simulink library "dsc"  (R2021b)
settings: Solver=VariableStepAuto  StartTime=0.0  StopTime=10.0  RelTol=1e-3
undefined symbols (not defined in the file): DEG2RAD, ENUM_DISCSTA_ACTIVE, ENUM_DISCSTA_Disabled, ENUM_DISCSTA_OFF, ENUM_DISCSTA_STANDBY, FALSE, KDSC_AccPedalOvrd_flg, KDSC_ActiveAllowTime_s, KDSC_BrkDisBand_pct, KDSC_BrkEnBand_pct, KDSC_BrkPedalOvrd_flg, KDSC_CGRealAxle_m, KDSC_FirstOrderInpTs_s, KDSC_LongAccelLimit_g, KDSC_MaxSpeed_kph, KDSC_MinSpeed_kph, KDSC_SamplingTime_s, KDSC_SpdRangeHigh_kph, KDSC_SpdRangeLow_kph, KDSC_TriggerTimes, KDSC_TurnAngControlpoint1_deg, KDSC_TurnAngControlpoint1_kph, KDSC_TurnAngControlpoint2_deg, KDSC_TurnAngControlpoint2_kph, KDSC_TurnAngExit_deg, KDSC_TurnAngLimit_deg, KINP_DISCButtReq_flg_ovrdflg, KINP_DISCButtReq_flg_ovrdval, RAD2DEG, TRUE, ZERO_FLOAT
libraries: simulink x13, hcu_lib x2
settings Model: Creator=FVT22120  LastModifiedBy=FVT23010

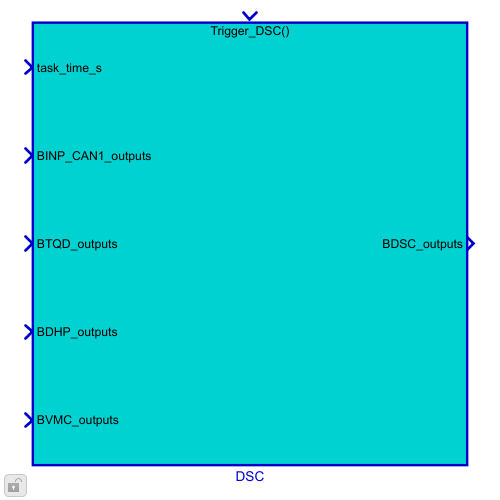
[thumbnail: Simulink's stored preview of the top-level diagram]
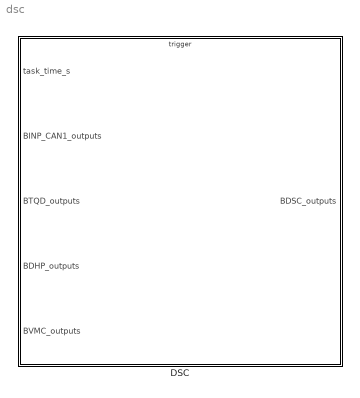
== system dsc ==
  DSC : Subsystem
      settings: RTWSystemCode=Nonreusable function  RTWFcnNameOpts=Use subsystem name  RTWFileNameOpts=Use subsystem name

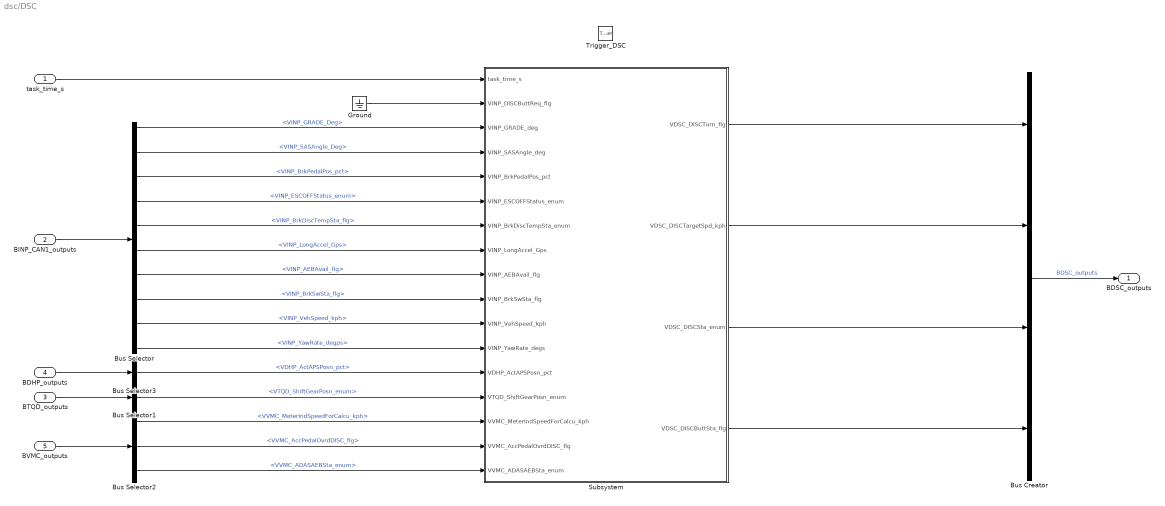
== system dsc/DSC ==
  task_time_s : Inport
  BINP_CAN1_outputs : Inport  Port=2  OutDataTypeStr=Bus: BINP_CAN1_outputs
  BTQD_outputs : Inport  Port=3  OutDataTypeStr=Bus: BTQD_outputs
  BDHP_outputs : Inport  Port=4  OutDataTypeStr=Bus: BDHP_outputs
  BVMC_outputs : Inport  Port=5  OutDataTypeStr=Bus: BVMC_outputs
  Trigger_DSC : TriggerPort  TriggerType=function-call  VariantControl=(inherit)  PortDimensions=1
  Bus Creator : BusCreator  Inputs=4  OutDataTypeStr=Bus: BDSC_outputs  NonVirtualBus=on
  Bus Selector : BusSelector  OutputSignals=VINP_GRADE_Deg,VINP_SASAngle_Deg,VINP_BrkPedalPos_pct,VINP_ESCOFFStatus_enum,VINP_BrkDiscTempSta_flg,VINP_LongAccel_Gps,VINP_AEBAvail_flg,VINP_BrkSwSta_flg,VINP_VehSpeed_kph,VINP_YawRate_degps
  Bus Selector1 : BusSelector  OutputSignals=VTQD_ShiftGearPosn_enum
  Bus Selector2 : BusSelector  OutputSignals=VVMC_MeterIndSpeedForCalcu_kph,VVMC_AccPedalOvrdDISC_flg,VVMC_ADASAEBSta_enum
  Bus Selector3 : BusSelector  OutputSignals=VDHP_ActAPSPosn_pct
  Ground : Ground
  Subsystem : Subsystem
  BDSC_outputs : Outport  OutDataTypeStr=Bus: BDSC_outputs
  wires:
  Bus Creator/1 -> BDSC_outputs/1  "BDSC_outputs"
  BINP_CAN1_outputs/1 -> Bus Selector/1
  BTQD_outputs/1 -> Bus Selector1/1
  BDHP_outputs/1 -> Bus Selector3/1
  task_time_s/1 -> Subsystem/1(task_time_s)
  Ground/1 -> Subsystem/2(VINP_DISCButtReq_flg)
  Bus Selector2/3 -> Subsystem/17(VVMC_ADASAEBSta_enum)  "<VVMC_ADASAEBSta_enum>"
  Bus Selector1/1 -> Subsystem/14(VTQD_ShiftGearPosn_enum)  "<VTQD_ShiftGearPosn_enum>"
  Bus Selector3/1 -> Subsystem/13(VDHP_ActAPSPosn_pct)  "<VDHP_ActAPSPosn_pct>"
  Subsystem/1(VDSC_DISCTurn_flg) -> Bus Creator/1
  Subsystem/2(VDSC_DISCTargetSpd_kph) -> Bus Creator/2
  Subsystem/3(VDSC_DISCSta_enum) -> Bus Creator/3
  Subsystem/4(VDSC_DISCButtSta_flg) -> Bus Creator/4
  BVMC_outputs/1 -> Bus Selector2/1
  Bus Selector2/1 -> Subsystem/15(VVMC_MeterIndSpeedForCalcu_kph)  "<VVMC_MeterIndSpeedForCalcu_kph>"
  Bus Selector2/2 -> Subsystem/16(VVMC_AccPedalOvrdDISC_flg)  "<VVMC_AccPedalOvrdDISC_flg>"
  Bus Selector/1 -> Subsystem/3(VINP_GRADE_deg)  "<VINP_GRADE_Deg>"
  Bus Selector/2 -> Subsystem/4(VINP_SASAngle_deg)  "<VINP_SASAngle_Deg>"
  Bus Selector/3 -> Subsystem/5(VINP_BrkPedalPos_pct)  "<VINP_BrkPedalPos_pct>"
  Bus Selector/4 -> Subsystem/6(VINP_ESCOFFStatus_enum)  "<VINP_ESCOFFStatus_enum>"
  Bus Selector/5 -> Subsystem/7(VINP_BrkDiscTempSta_enum)  "<VINP_BrkDiscTempSta_flg>"
  Bus Selector/6 -> Subsystem/8(VINP_LongAccel_Gps)  "<VINP_LongAccel_Gps>"
  Bus Selector/7 -> Subsystem/9(VINP_AEBAvail_flg)  "<VINP_AEBAvail_flg>"
  Bus Selector/8 -> Subsystem/10(VINP_BrkSwSta_flg)  "<VINP_BrkSwSta_flg>"
  Bus Selector/9 -> Subsystem/11(VINP_VehSpeed_kph)  "<VINP_VehSpeed_kph>"
  Bus Selector/10 -> Subsystem/12(VINP_YawRate_degs)  "<VINP_YawRate_degps>"

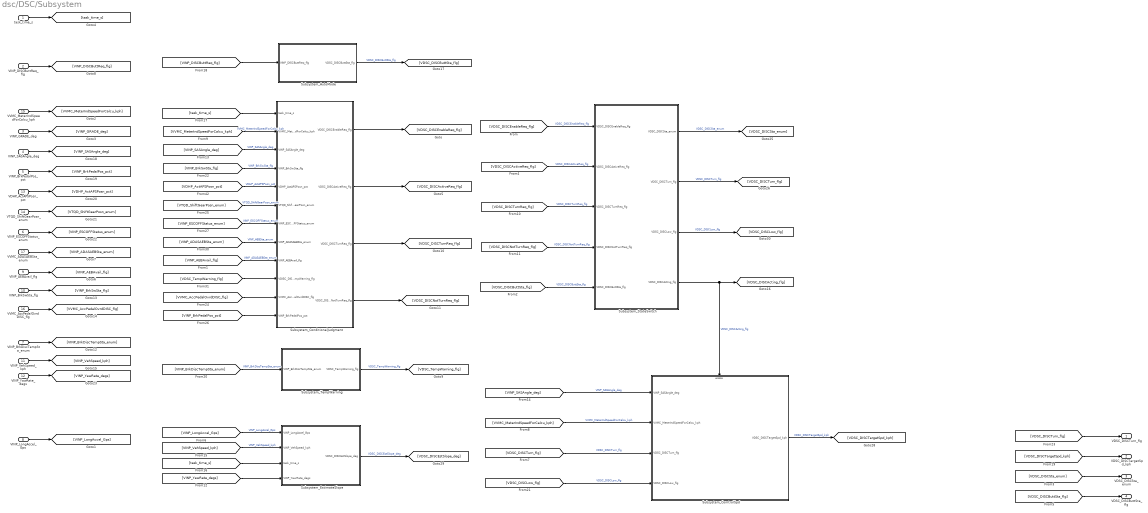
== system dsc/DSC/Subsystem ==
  task_time_s : Inport
  VINP_DISCButtReq_flg : Inport  Port=2
  VINP_GRADE_deg : Inport  Port=3
  VINP_SASAngle_deg : Inport  Port=4
  VINP_BrkPedalPos_pct : Inport  Port=5
  VINP_ESCOFFStatus_enum : Inport  Port=6
  VINP_BrkDiscTempSta_enum : Inport  Port=7
  VINP_LongAccel_Gps : Inport  Port=8
  VINP_AEBAvail_flg : Inport  Port=9
  VINP_BrkSwSta_flg : Inport  Port=10
  VINP_VehSpeed_kph : Inport  Port=11
  VINP_YawRate_degs : Inport  Port=12
  VDHP_ActAPSPosn_pct : Inport  Port=13
  VTQD_ShiftGearPosn_enum : Inport  Port=14
  VVMC_MeterIndSpeedForCalcu_kph : Inport  Port=15
  VVMC_AccPedalOvrdDISC_flg : Inport  Port=16
  VVMC_ADASAEBSta_enum : Inport  Port=17
  Subsystem_AutoMode : Subsystem
  Subsystem_ComtrolSpd : Subsystem  TreatAsAtomicUnit=on
  Subsystem_ConditionalJudgment : Subsystem
  Subsystem_EstimateSlope : Subsystem
  Subsystem_StateSwitch : Subsystem
  Subsystem_TempWarning : Subsystem
  VDSC_DISCTurn_flg : Outport
  VDSC_DISCTargetSpd_kph : Outport  Port=2
  VDSC_DISCSta_enum : Outport  Port=3
  VDSC_DISCButtSta_flg : Outport  Port=4
  wires:
  Subsystem_StateSwitch/4(VDSC_DISCActing_flg) -> [VDSC_DISCActing_flg], Subsystem_ComtrolSpd/Enable  "VDSC_DISCActing_flg"
  [VINP_SASAngle_deg] -> Subsystem_ConditionalJudgment/3("VINP_SASAngle_deg ")  "VINP_SASAngle_deg"
  [VDSC_DISCEnableReq_flg] -> Subsystem_StateSwitch/1(VDSC_DISCEnableReq_flg)  "VDSC_DISCEnableReq_flg"
  Subsystem_StateSwitch/2(VDSC_DISCTurn_flg) -> [VDSC_DISCTurn_flg]  "VDSC_DISCTurn_flg"
  [VINP_VehSpeed_kph] -> Subsystem_EstimateSlope/2(VINP_VehSpeed_kph)  "VINP_VehSpeed_kph"
  [VINP_DISCButtReq_flg] -> Subsystem_AutoMode/1(VINP_DISCButtReq_flg)
  VINP_GRADE_deg/1 -> [VINP_GRADE_deg]
  Subsystem_EstimateSlope/1(VDSC_DISCEstSlope_deg) -> [VDSC_DISCEstSlope_deg]  "VDSC_DISCEstSlope_deg"
  VTQD_ShiftGearPosn_enum/1 -> [VTQD_ShiftGearPosn_enum]
  Subsystem_ConditionalJudgment/3(VDSC_DISCTurnReq_flg) -> [VDSC_DISCTurnReq_flg]
  [VDSC_DISCTurn_flg] -> Subsystem_ComtrolSpd/3(VDSC_DISCTurn_flg)  "VDSC_DISCTurn_flg"
  VINP_LongAccel_Gps/1 -> [VINP_LongAccel_Gps]
  [VDSC_DISCTargetSpd_kph] -> VDSC_DISCTargetSpd_kph/1
  [VDSC_DISCButtSta_flg] -> VDSC_DISCButtSta_flg/1
  [VINP_LongAccel_Gps] -> Subsystem_EstimateSlope/1(VINP_LongAccel_Gps)  "VINP_LongAccel_Gps"
  Subsystem_AutoMode/1(VDSC_DISCButtSta_flg) -> [VDSC_DISCButtSta_flg]  "VDSC_DISCButtSta_flg"
  VINP_SASAngle_deg/1 -> [VINP_SASAngle_deg]
  VINP_AEBAvail_flg/1 -> [VINP_AEBAvail_flg]
  [VDSC_TempWarning_flg] -> Subsystem_ConditionalJudgment/10(VDISC_DISCTempWarning_flg)
  Subsystem_ComtrolSpd/1(VDSC_DISCTargetSpd_kph) -> [VDSC_DISCTargetSpd_kph]  "VDSC_DISCTargetSpd_kph"
  [VDSC_DISCTurn_flg] -> VDSC_DISCTurn_flg/1
  VVMC_ADASAEBSta_enum/1 -> [VINP_ADASAEBSta_enum]
  [VVMC_MeterIndSpeedForCalcu_kph] -> Subsystem_ComtrolSpd/2(VVMC_MeterIndSpeedForCalcu_kph)  "VVMC_MeterIndSpeedForCalcu_kph"
  [VDSC_DISCActiveReq_flg] -> Subsystem_StateSwitch/2(VDSC_DISCActiveReq_flg)  "VDSC_DISCActiveReq_flg"
  VINP_BrkSwSta_flg/1 -> [VINP_BrkSwSta_flg]
  [VINP_BrkPedalPos_pct] -> Subsystem_ConditionalJudgment/12(VINP_BrkPedalPos_pct)
  VVMC_AccPedalOvrdDISC_flg/1 -> [VVMC_AccPedalOvrdDISC_flg]
  VDHP_ActAPSPosn_pct/1 -> [VDHP_ActAPSPosn_pct]
  [task_time_s] -> Subsystem_EstimateSlope/3(task_time_s)
  [task_time_s] -> Subsystem_ConditionalJudgment/1(task_time_s)
  VINP_BrkDiscTempSta_enum/1 -> [VINP_BrkDiscTempSta_enum]
  [VVMC_AccPedalOvrdDISC_flg] -> Subsystem_ConditionalJudgment/11(VVMC_AccPedalOvrdDISC_flg)
  VINP_VehSpeed_kph/1 -> [VINP_VehSpeed_kph]
  Subsystem_ConditionalJudgment/4(VDSC_DISCNotTurnReq_flg) -> [VDSC_DISCNotTurnReq_flg]
  [VDHP_ActAPSPosn_pct] -> Subsystem_ConditionalJudgment/5("VDHP_ActAPSPosn_pct ")  "VDHP_ActAPSPosn_pct"
  [VDSC_DISCNotTurnReq_flg] -> Subsystem_StateSwitch/4(VDSC_DISCNotTurnReq_flg)  "VDSC_DISCNotTurnReq_flg"
  [VINP_AEBAvail_flg] -> Subsystem_ConditionalJudgment/9(VINP_AEBAvail_flg)  "VINP_ADASAEBSta_enum"
  Subsystem_ConditionalJudgment/1(VDSC_DISCEnableReq_flg) -> [VDSC_DISCEnableReq_flg]
  Subsystem_StateSwitch/1(VDSC_DISCSta_enum) -> [VDSC_DISCSta_enum]  "VDSC_DISCSta_enum"
  [VINP_SASAngle_deg] -> Subsystem_ComtrolSpd/1(VINP_SASAngle_deg)  "VINP_SASAngle_deg"
  VINP_BrkPedalPos_pct/1 -> [VINP_BrkPedalPos_pct]
  VINP_DISCButtReq_flg/1 -> [VINP_DISCButtReq_flg]
  VINP_ESCOFFStatus_enum/1 -> [VINP_ESCOFFStatus_enum]
  VVMC_MeterIndSpeedForCalcu_kph/1 -> [VVMC_MeterIndSpeedForCalcu_kph]
  [VINP_ADASAEBSta_enum] -> Subsystem_ConditionalJudgment/8(VINP_ADASAEBSta_enum)  "VINP_AEBSta_enum"
  [VINP_BrkDiscTempSta_enum] -> Subsystem_TempWarning/1(VINP_BrkDiscTempSta_enum)  "VINP_BrkDiscTempSta_enum"
  Subsystem_ConditionalJudgment/2(VDSC_DISCActiveReq_flg) -> [VDSC_DISCActiveReq_flg]
  [VTQD_ShiftGearPosn_enum] -> Subsystem_ConditionalJudgment/6("VTQD_ShiftGearPosn_enum ")  "VTQD_ShiftGearPosn_enum"
  [VVMC_MeterIndSpeedForCalcu_kph] -> Subsystem_ConditionalJudgment/2("VVMC_MeterIndSpeedForCalcu_kph ")  "VVMC_MeterIndSpeedForCalcu_kph"
  [VDSC_DISCLow_flg] -> Subsystem_ComtrolSpd/4(VDSC_DISCLow_flg)  "VDSC_DISCLow_flg"
  [VINP_ESCOFFStatus_enum] -> Subsystem_ConditionalJudgment/7(VINP_ESCOFFStatus_enum)  "VINP_ESCOFFStatus_enum"
  task_time_s/1 -> [task_time_s]
  [VDSC_DISCButtSta_flg] -> Subsystem_StateSwitch/5(VDSC_DISCButtSta_flg)  "VDSC_DISCButtSta_flg"
  Subsystem_StateSwitch/3(VDSC_DISCLow_flg) -> [VDSC_DISCLow_flg]  "VDSC_DISCLow_flg"
  Subsystem_TempWarning/1(VDSC_TempWarning_flg) -> [VDSC_TempWarning_flg]  "VDSC_TempWarning_flg"
  [VDSC_DISCSta_enum] -> VDSC_DISCSta_enum/1
  [VINP_BrkSwSta_flg] -> Subsystem_ConditionalJudgment/4("VINP_BrkSwSta_flg ")  "VINP_BrkSwSta_flg"
  [VDSC_DISCTurnReq_flg] -> Subsystem_StateSwitch/3(VDSC_DISCTurnReq_flg)  "VDSC_DISCTurnReq_flg"
  VINP_YawRate_degs/1 -> [VINP_YawRate_degs]
  [VINP_YawRate_degs] -> Subsystem_EstimateSlope/4(VINP_YawRate_degs)

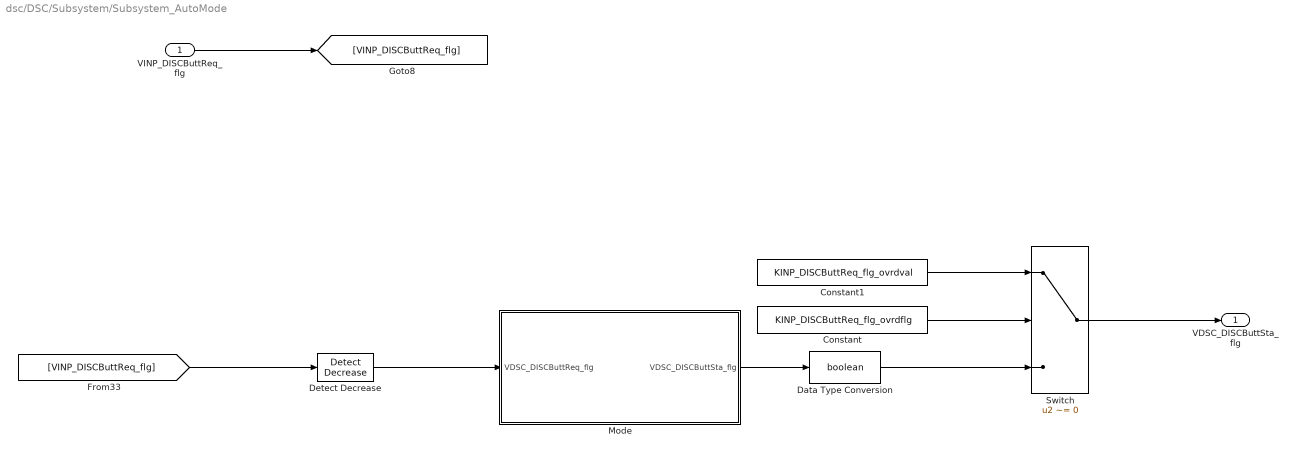
== system dsc/DSC/Subsystem/Subsystem_AutoMode ==
  VINP_DISCButtReq_flg : Inport
  Constant : Constant  Value=KINP_DISCButtReq_flg_ovrdflg
  Constant1 : Constant  Value=KINP_DISCButtReq_flg_ovrdval
  Data Type Conversion : DataTypeConversion  OutDataTypeStr=boolean
  Detect Decrease : simulink/Logic and Bit Operations/Detect Decrease  vinit=0.0  OutDataTypeStr=boolean
  Mode : Stateflow chart  TreatAsAtomicUnit=on
  Switch : Switch  Criteria=u2 ~= 0
  VDSC_DISCButtSta_flg : Outport
  wires:
  Mode/1(VDSC_DISCButtSta_flg) -> Data Type Conversion/1
  VINP_DISCButtReq_flg/1 -> [VINP_DISCButtReq_flg]
  Detect Decrease/1 -> Mode/1(VDSC_DISCButtReq_flg)
  Data Type Conversion/1 -> Switch/3
  [VINP_DISCButtReq_flg] -> Detect Decrease/1
  Constant/1 -> Switch/2
  Constant1/1 -> Switch/1
  Switch/1 -> VDSC_DISCButtSta_flg/1

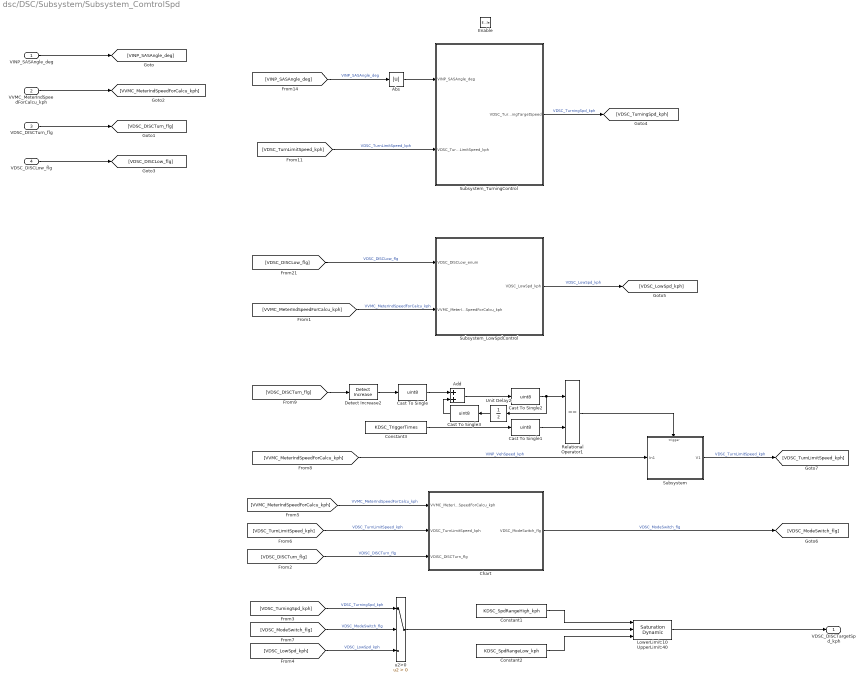
== system dsc/DSC/Subsystem/Subsystem_ComtrolSpd ==
  VINP_SASAngle_deg : Inport
  VVMC_MeterIndSpeedForCalcu_kph : Inport  Port=2
  VDSC_DISCTurn_flg : Inport  Port=3
  VDSC_DISCLow_flg : Inport  Port=4
  Enable : EnablePort  StatesWhenEnabling=reset
  Abs : Abs
  Add : Sum
  Cast To Single{,1..3} (4 alike) : DataTypeConversion  OutDataTypeStr=uint8
  Chart : Stateflow chart  TreatAsAtomicUnit=on
  Constant1 : Constant  Value=KDSC_SpdRangeHigh_kph
  Constant2 : Constant  Value=KDSC_SpdRangeLow_kph
  Constant3 : Constant  Value=KDSC_TriggerTimes
  Detect Increase2 : simulink/Logic and Bit Operations/Detect Increase  vinit=0.0  OutDataTypeStr=boolean
  LowerLimit:10 UpperLimit:40 : simulink/Discontinuities/Saturation Dynamic  OutMin=[]  OutMax=[]  OutDataTypeStr=Inherit: Same as second input  OutDataType=fixdt(1, 16)  OutScaling=2^-10  DoSatur=off
  Relational Operator1 : RelationalOperator  Operator===  OutDataTypeStr=boolean  RndMeth=Simplest
  Subsystem : Subsystem
  Subsystem_LowSpdControl : Subsystem
  Subsystem_TurningControl : Subsystem  TreatAsAtomicUnit=on
  Unit Delay2 : UnitDelay  SampleTime=-1  HasFrameUpgradeWarning=on
  u2>0 : Switch  Criteria=u2 > Threshold  OutDataTypeStr=single
  VDSC_DISCTargetSpd_kph : Outport
  wires:
  Subsystem_LowSpdControl/1(VDSC_LowSpd_kph) -> [VDSC_LowSpd_kph]  "VDSC_LowSpd_kph"
  [VDSC_ModeSwitch_flg] -> u2>0/2  "VDSC_ModeSwitch_flg"
  Constant1/1 -> LowerLimit:10 UpperLimit:40/1
  Constant2/1 -> LowerLimit:10 UpperLimit:40/3
  Abs/1 -> Subsystem_TurningControl/1(VINP_SASAngle_deg)
  Subsystem_TurningControl/1(VDSC_TurningTargetSpeed) -> [VDSC_TurningSpd_kph]  "VDSC_TurningSpd_kph"
  u2>0/1 -> LowerLimit:10 UpperLimit:40/2
  [VDSC_DISCLow_flg] -> Subsystem_LowSpdControl/1(VDSC_DISCLow_enum)  "VDSC_DISCLow_flg"
  VINP_SASAngle_deg/1 -> [VINP_SASAngle_deg]
  [VINP_SASAngle_deg] -> Abs/1  "VINP_SASAngle_deg"
  VVMC_MeterIndSpeedForCalcu_kph/1 -> [VVMC_MeterIndSpeedForCalcu_kph]
  [VVMC_MeterIndSpeedForCalcu_kph] -> Subsystem_LowSpdControl/2(VVMC_MeterIndSpeedForCalcu_kph)  "VVMC_MeterIndSpeedForCalcu_kph"
  VDSC_DISCTurn_flg/1 -> [VDSC_DISCTurn_flg]
  VDSC_DISCLow_flg/1 -> [VDSC_DISCLow_flg]
  [VDSC_TurningSpd_kph] -> u2>0/1  "VDSC_TurningSpd_kph"
  [VDSC_LowSpd_kph] -> u2>0/3  "VDSC_LowSpd_kph"
  LowerLimit:10 UpperLimit:40/1 -> VDSC_DISCTargetSpd_kph/1
  [VDSC_DISCTurn_flg] -> Detect Increase2/1
  Chart/1(VDSC_ModeSwitch_flg) -> [VDSC_ModeSwitch_flg]  "VDSC_ModeSwitch_flg"
  Constant3/1 -> Cast To Single1/1
  Relational Operator1/1 -> Subsystem/Trigger
  Subsystem/1(V1) -> [VDSC_TurnLimitSpeed_kph]  "VDSC_TurnLimitSpeed_kph"
  Detect Increase2/1 -> Cast To Single/1
  [VDSC_DISCTurn_flg] -> Chart/3(VDISC_DISCTurn_flg)  "VDISC_DISCTurn_flg"
  [VDSC_TurnLimitSpeed_kph] -> Chart/2(VDSC_TurnLimitSpeed_kph)  "VDSC_TurnLimitSpeed_kph"
  [VVMC_MeterIndSpeedForCalcu_kph] -> Subsystem/1(In1)  "VINP_VehSpeed_kph"
  [VVMC_MeterIndSpeedForCalcu_kph] -> Chart/1(VVMC_MeterIndSpeedForCalcu_kph)  "VVMC_MeterIndSpeedForCalcu_kph"
  [VDSC_TurnLimitSpeed_kph] -> Subsystem_TurningControl/2(VDSC_TurnLimitSpeed_kph)  "VDSC_TurnLimitSpeed_kph"
  Add/1 -> Cast To Single2/1
  Unit Delay2/1 -> Cast To Single3/1
  Cast To Single/1 -> Add/1
  Cast To Single1/1 -> Relational Operator1/2
  Cast To Single2/1 -> Unit Delay2/1, Relational Operator1/1
  Cast To Single3/1 -> Add/2

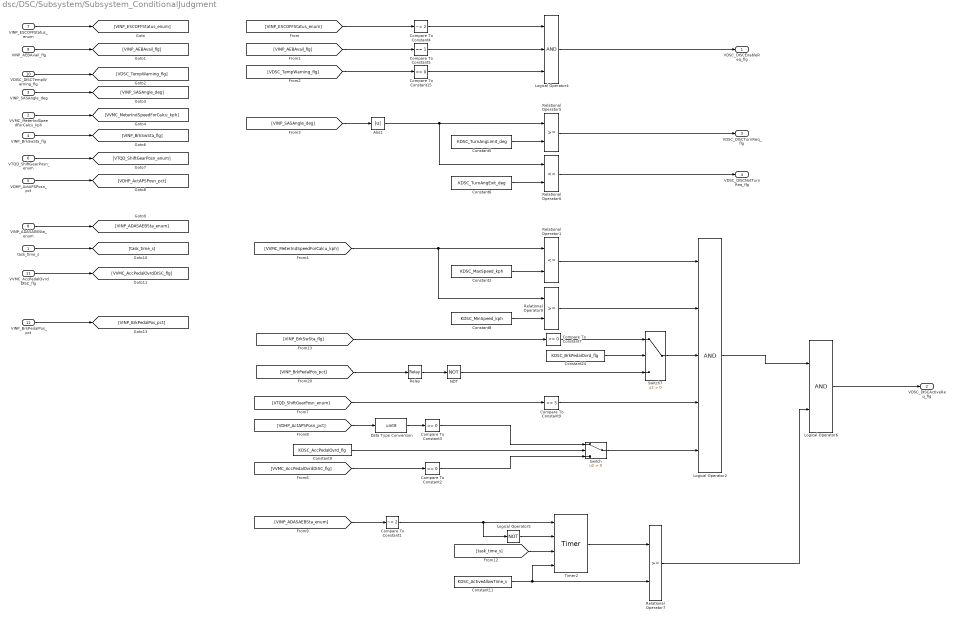
== system dsc/DSC/Subsystem/Subsystem_ConditionalJudgment ==
  task_time_s : Inport
  "VVMC_MeterIndSpeedForCalcu_kph " : Inport  Port=2
  "VINP_SASAngle_deg " : Inport  Port=3
  "VINP_BrkSwSta_flg " : Inport  Port=4
  "VDHP_ActAPSPosn_pct " : Inport  Port=5
  "VTQD_ShiftGearPosn_enum " : Inport  Port=6
  VINP_ESCOFFStatus_enum : Inport  Port=7
  VINP_ADASAEBSta_enum : Inport  Port=8
  VINP_AEBAvail_flg : Inport  Port=9
  VDISC_DISCTempWarning_flg : Inport  Port=10
  VVMC_AccPedalOvrdDISC_flg : Inport  Port=11
  VINP_BrkPedalPos_pct : Inport  Port=12
  Abs2 : Abs
  Compare To Constant1 : simulink/Logic and Bit Operations/Compare To Constant  relop=~=  const=2  OutDataTypeStr=boolean
  Compare To Constant{2..3,7,15} (4 alike) : simulink/Logic and Bit Operations/Compare To Constant  relop===  const=0  OutDataTypeStr=boolean
  Compare To Constant4 : simulink/Logic and Bit Operations/Compare To Constant  relop=~=  const=2  OutDataTypeStr=boolean
  Compare To Constant5 : simulink/Logic and Bit Operations/Compare To Constant  relop===  const=1  OutDataTypeStr=boolean
  Compare To Constant9 : simulink/Logic and Bit Operations/Compare To Constant  relop===  const=5  OutDataTypeStr=boolean
  Constant11 : Constant  Value=KDSC_ActiveAllowTime_s
  Constant2 : Constant  Value=KDSC_MaxSpeed_kph
  Constant24 : Constant  Value=KDSC_BrkPedalOvrd_flg
  Constant5 : Constant  Value=KDSC_TurnAngLimit_deg
  Constant6 : Constant  Value=KDSC_TurnAngExit_deg
  Constant8 : Constant  Value=KDSC_MinSpeed_kph
  Constant9 : Constant  Value=KDSC_AccPedalOvrd_flg
  Data Type Conversion : DataTypeConversion  OutDataTypeStr=uint8
  Logical Operator2 : Logic  Inputs=5  AllPortsSameDT=off  OutDataTypeStr=boolean
  Logical Operator4 : Logic  Inputs=3  AllPortsSameDT=off  OutDataTypeStr=boolean
  Logical Operator5 : Logic  Operator=NOT  Inputs=6  AllPortsSameDT=off  OutDataTypeStr=boolean
  Logical Operator6 : Logic  AllPortsSameDT=off  OutDataTypeStr=boolean
  NOT : Logic  Operator=NOT  AllPortsSameDT=off  OutDataTypeStr=boolean
  Relational Operator1 : RelationalOperator  Operator=<=  OutDataTypeStr=boolean  RndMeth=Simplest
  Relational Operator5 : RelationalOperator  OutDataTypeStr=boolean  RndMeth=Simplest
  Relational Operator6 : RelationalOperator  Operator=<=  OutDataTypeStr=boolean  RndMeth=Simplest
  Relational Operator7 : RelationalOperator  OutDataTypeStr=boolean  RndMeth=Simplest
  Relational Operator9 : RelationalOperator  OutDataTypeStr=boolean  RndMeth=Simplest
  Relay : Relay  OnSwitchValue=KDSC_BrkEnBand_pct  OffSwitchValue=KDSC_BrkDisBand_pct
  Switch : Switch  Criteria=u2 > Threshold
  Switch7 : Switch  Criteria=u2 > Threshold
  Timer2 : hcu_lib/Basic_Blocks/Timer
  VDSC_DISCEnableReq_flg : Outport
  VDSC_DISCActiveReq_flg : Outport  Port=2
  VDSC_DISCTurnReq_flg : Outport  Port=3
  VDSC_DISCNotTurnReq_flg : Outport  Port=4
  wires:
  Logical Operator2/1 -> Logical Operator6/1
  [VTQD_ShiftGearPosn_enum] -> Compare To Constant9/1
  Compare To Constant3/1 -> Switch/1
  Compare To Constant9/1 -> Logical Operator2/4
  Compare To Constant7/1 -> Switch7/1
  [VDHP_ActAPSPosn_pct] -> Data Type Conversion/1
  VDISC_DISCTempWarning_flg/1 -> [VDSC_TempWarning_flg]
  Relational Operator9/1 -> Logical Operator2/2
  "VVMC_MeterIndSpeedForCalcu_kph "/1 -> [VVMC_MeterIndSpeedForCalcu_kph]
  [VINP_SASAngle_deg] -> Abs2/1
  "VINP_BrkSwSta_flg "/1 -> [VINP_BrkSwSta_flg]
  [VDSC_TempWarning_flg] -> Compare To Constant15/1
  [VINP_AEBAvail_flg] -> Compare To Constant5/1
  Constant5/1 -> Relational Operator5/2
  Relational Operator1/1 -> Logical Operator2/1
  Compare To Constant5/1 -> Logical Operator4/2
  Constant2/1 -> Relational Operator1/2
  Compare To Constant15/1 -> Logical Operator4/3
  Relational Operator6/1 -> VDSC_DISCNotTurnReq_flg/1
  Compare To Constant1/1 -> Logical Operator5/1, Timer2/1
  Compare To Constant4/1 -> Logical Operator4/1
  Constant11/1 -> Timer2/4, Relational Operator7/2
  VINP_AEBAvail_flg/1 -> [VINP_AEBAvail_flg]
  Relational Operator5/1 -> VDSC_DISCTurnReq_flg/1
  [VINP_ESCOFFStatus_enum] -> Compare To Constant4/1
  Abs2/1 -> Relational Operator5/1, Relational Operator6/1
  [task_time_s] -> Timer2/3
  "VTQD_ShiftGearPosn_enum "/1 -> [VTQD_ShiftGearPosn_enum]
  [VINP_ADASAEBSta_enum] -> Compare To Constant1/1
  Constant6/1 -> Relational Operator6/2
  Constant8/1 -> Relational Operator9/2
  [VINP_BrkSwSta_flg] -> Compare To Constant7/1
  Logical Operator5/1 -> Timer2/2
  "VDHP_ActAPSPosn_pct "/1 -> [VDHP_ActAPSPosn_pct]
  VINP_ESCOFFStatus_enum/1 -> [VINP_ESCOFFStatus_enum]
  [VVMC_MeterIndSpeedForCalcu_kph] -> Relational Operator9/1, Relational Operator1/1
  Logical Operator4/1 -> VDSC_DISCEnableReq_flg/1
  Logical Operator6/1 -> VDSC_DISCActiveReq_flg/1
  VINP_ADASAEBSta_enum/1 -> [VINP_ADASAEBSta_enum]
  Relational Operator7/1 -> Logical Operator6/2
  "VINP_SASAngle_deg "/1 -> [VINP_SASAngle_deg]
  task_time_s/1 -> [task_time_s]
  Timer2/1 -> Relational Operator7/1
  VVMC_AccPedalOvrdDISC_flg/1 -> [VVMC_AccPedalOvrdDISC_flg]
  [VVMC_AccPedalOvrdDISC_flg] -> Compare To Constant2/1
  Switch/1 -> Logical Operator2/5
  Constant9/1 -> Switch/2
  Compare To Constant2/1 -> Switch/3
  Constant24/1 -> Switch7/2
  Switch7/1 -> Logical Operator2/3
  VINP_BrkPedalPos_pct/1 -> [VINP_BrkPedalPos_pct]
  [VINP_BrkPedalPos_pct] -> Relay/1
  Relay/1 -> NOT/1
  NOT/1 -> Switch7/3
  Data Type Conversion/1 -> Compare To Constant3/1

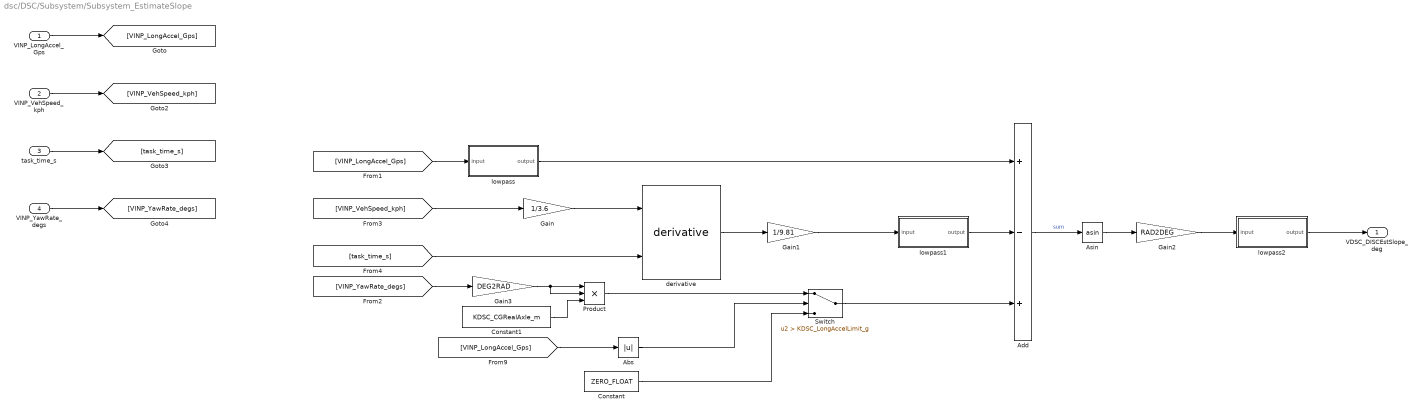
== system dsc/DSC/Subsystem/Subsystem_EstimateSlope ==
  VINP_LongAccel_Gps : Inport
  VINP_VehSpeed_kph : Inport  Port=2
  task_time_s : Inport  Port=3
  VINP_YawRate_degs : Inport  Port=4
  Abs : Abs
  Add : Sum  Inputs=+-+
  Asin : Trigonometry  Operator=asin
  Constant : Constant  Value=ZERO_FLOAT
  Constant1 : Constant  Value=KDSC_CGRealAxle_m
  Gain : Gain  Gain=1/3.6
  Gain1 : Gain  Gain=1/9.81
  Gain2 : Gain  Gain=RAD2DEG
  Gain3 : Gain  Gain=DEG2RAD
  Product : Product  Inputs=3
  Switch : Switch  Criteria=u2 > Threshold  Threshold=KDSC_LongAccelLimit_g
  derivative : hcu_lib/Basic_Blocks/derivative
  lowpass : Subsystem
  lowpass1 : Subsystem
  lowpass2 : Subsystem
  VDSC_DISCEstSlope_deg : Outport
  wires:
  Gain/1 -> derivative/1
  Gain1/1 -> lowpass1/1(input)
  Add/1 -> Asin/1  "sum"
  lowpass/1(output) -> Add/1
  [VINP_VehSpeed_kph] -> Gain/1
  derivative/1 -> Gain1/1
  lowpass2/1(output) -> VDSC_DISCEstSlope_deg/1
  Asin/1 -> Gain2/1
  Gain2/1 -> lowpass2/1(input)
  VINP_LongAccel_Gps/1 -> [VINP_LongAccel_Gps]
  [VINP_LongAccel_Gps] -> lowpass/1(input)
  [VINP_LongAccel_Gps] -> Abs/1
  Abs/1 -> Switch/2
  VINP_VehSpeed_kph/1 -> [VINP_VehSpeed_kph]
  task_time_s/1 -> [task_time_s]
  [task_time_s] -> derivative/2
  VINP_YawRate_degs/1 -> [VINP_YawRate_degs]
  [VINP_YawRate_degs] -> Gain3/1
  Constant/1 -> Switch/3
  Switch/1 -> Add/3
  Gain3/1 -> Product/2, Product/1
  lowpass1/1(output) -> Add/2
  Product/1 -> Switch/1
  Constant1/1 -> Product/3

== system dsc/DSC/Subsystem/Subsystem_StateSwitch ==
  VDSC_DISCEnableReq_flg : Inport
  VDSC_DISCActiveReq_flg : Inport  Port=2
  VDSC_DISCTurnReq_flg : Inport  Port=3
  VDSC_DISCNotTurnReq_flg : Inport  Port=4
  VDSC_DISCButtSta_flg : Inport  Port=5
  Chart1 : Stateflow chart  TreatAsAtomicUnit=on
  VDSC_DISCSta_enum : Outport
  VDSC_DISCTurn_flg : Outport  Port=2
  VDSC_DISCLow_flg : Outport  Port=3
  VDSC_DISCActing_flg : Outport  Port=4
  wires:
  VDSC_DISCEnableReq_flg/1 -> Chart1/1(VDSC_DISCEnableReq_flg)
  VDSC_DISCActiveReq_flg/1 -> Chart1/2(VDSC_DISCActiveReq_flg)
  VDSC_DISCTurnReq_flg/1 -> Chart1/3(VDSC_DISCTurnReq_flg)
  VDSC_DISCNotTurnReq_flg/1 -> Chart1/4(VDSC_DISCNotTurnReq_flg)
  VDSC_DISCButtSta_flg/1 -> Chart1/5(VDSC_DISCButtSta_flg)
  Chart1/1(VDSC_DISCSta_enum) -> VDSC_DISCSta_enum/1
  Chart1/2(VDSC_DISCTurn_flg) -> VDSC_DISCTurn_flg/1
  Chart1/3(VDSC_DISCLow_flg) -> VDSC_DISCLow_flg/1
  Chart1/4(VDSC_DISCActing_flg) -> VDSC_DISCActing_flg/1

== system dsc/DSC/Subsystem/Subsystem_TempWarning ==
  VINP_BrkDiscTempSta_enum : Inport
  Chart1 : Stateflow chart  TreatAsAtomicUnit=on
  VDSC_TempWarning_flg : Outport
  wires:
  [VINP_BrkDiscTempSta_enum] -> Chart1/1(VINP_BrkDiscTempSta_enum)
  VINP_BrkDiscTempSta_enum/1 -> [VINP_BrkDiscTempSta_enum]
  Chart1/1(VDSC_TempWarning_flg) -> VDSC_TempWarning_flg/1

== system dsc/DSC/Subsystem/Subsystem_ComtrolSpd/Subsystem ==
  In1 : Inport
  Trigger : TriggerPort  VariantControl=(inherit)  PortDimensions=1
  V1 : Outport
  wires:
  In1/1 -> V1/1

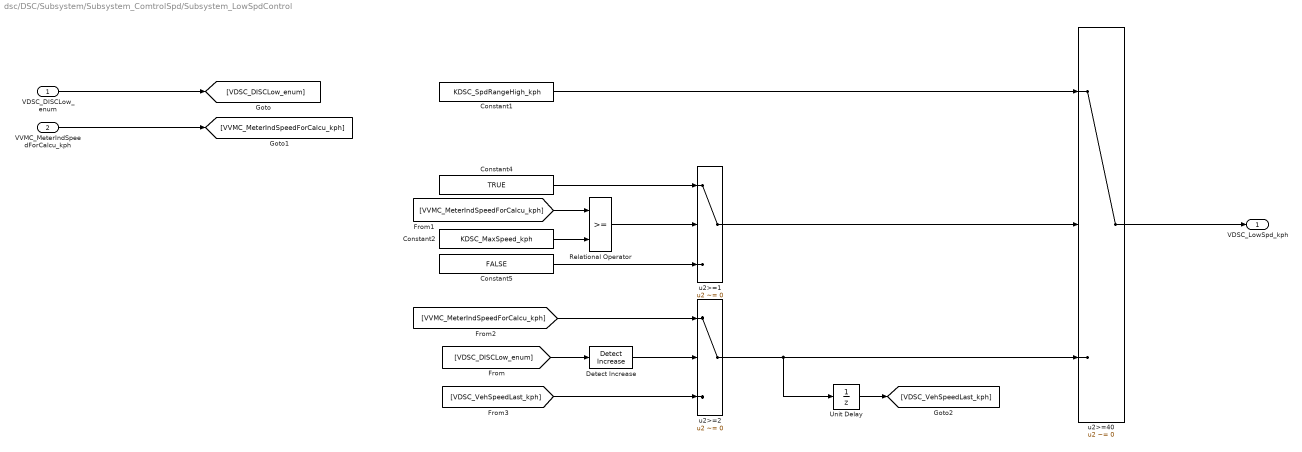
== system dsc/DSC/Subsystem/Subsystem_ComtrolSpd/Subsystem_LowSpdControl ==
  VDSC_DISCLow_enum : Inport
  VVMC_MeterIndSpeedForCalcu_kph : Inport  Port=2
  Constant1 : Constant  Value=KDSC_SpdRangeHigh_kph
  Constant2 : Constant  Value=KDSC_MaxSpeed_kph
  Constant4 : Constant  Value=TRUE
  Constant5 : Constant  Value=FALSE
  Detect Increase : simulink/Logic and Bit Operations/Detect Increase  vinit=0.0  OutDataTypeStr=boolean
  Relational Operator : RelationalOperator  OutDataTypeStr=boolean  RndMeth=Simplest
  Unit Delay : UnitDelay  SampleTime=-1  HasFrameUpgradeWarning=on
  u2>=1 : Switch  Criteria=u2 ~= 0
  u2>=2 : Switch  Criteria=u2 ~= 0
  u2>=40 : Switch  Criteria=u2 ~= 0
  VDSC_LowSpd_kph : Outport
  wires:
  [VDSC_DISCLow_enum] -> Detect Increase/1
  Constant1/1 -> u2>=40/1
  u2>=40/1 -> VDSC_LowSpd_kph/1
  VDSC_DISCLow_enum/1 -> [VDSC_DISCLow_enum]
  VVMC_MeterIndSpeedForCalcu_kph/1 -> [VVMC_MeterIndSpeedForCalcu_kph]
  Constant2/1 -> Relational Operator/2
  u2>=1/1 -> u2>=40/2
  Relational Operator/1 -> u2>=1/2
  [VVMC_MeterIndSpeedForCalcu_kph] -> Relational Operator/1
  Constant4/1 -> u2>=1/1
  Constant5/1 -> u2>=1/3
  Detect Increase/1 -> u2>=2/2
  [VVMC_MeterIndSpeedForCalcu_kph] -> u2>=2/1
  u2>=2/1 -> Unit Delay/1, u2>=40/3
  Unit Delay/1 -> [VDSC_VehSpeedLast_kph]
  [VDSC_VehSpeedLast_kph] -> u2>=2/3

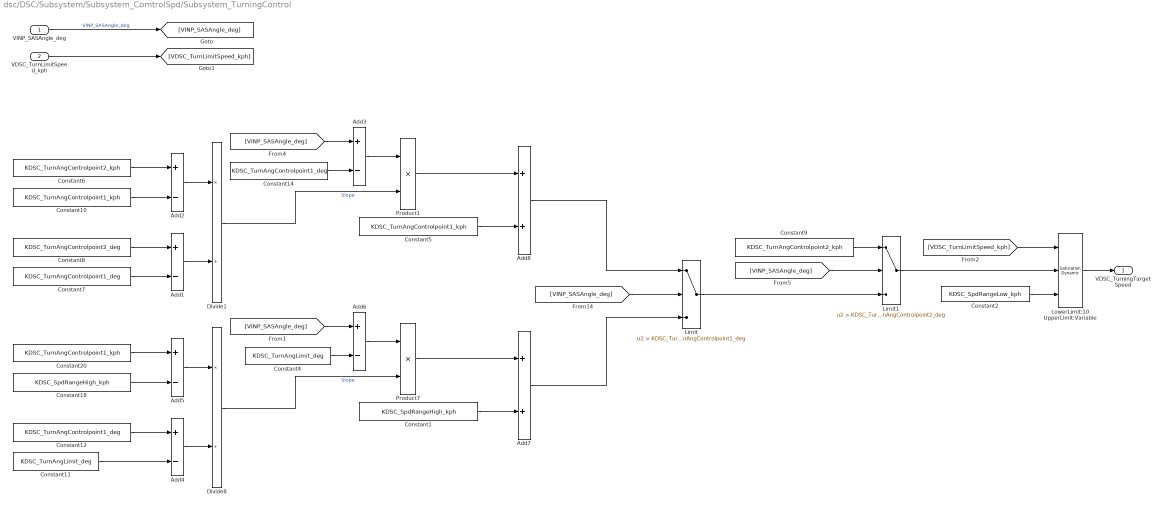
== system dsc/DSC/Subsystem/Subsystem_ComtrolSpd/Subsystem_TurningControl ==
  VINP_SASAngle_deg : Inport
  VDSC_TurnLimitSpeed_kph : Inport  Port=2
  Add{1..6} (6 alike) : Sum  Inputs=+-
  Add7 : Sum
  Add8 : Sum
  Constant1 : Constant  Value=KDSC_SpdRangeHigh_kph
  Constant10 : Constant  Value=KDSC_TurnAngControlpoint1_kph
  Constant11 : Constant  Value=KDSC_TurnAngLimit_deg
  Constant12 : Constant  Value=KDSC_TurnAngControlpoint1_deg
  Constant14 : Constant  Value=KDSC_TurnAngControlpoint1_deg
  Constant18 : Constant  Value=KDSC_SpdRangeHigh_kph
  Constant2 : Constant  Value=KDSC_SpdRangeLow_kph
  Constant20 : Constant  Value=KDSC_TurnAngControlpoint1_kph
  Constant4 : Constant  Value=KDSC_TurnAngLimit_deg
  Constant5 : Constant  Value=KDSC_TurnAngControlpoint1_kph
  Constant6 : Constant  Value=KDSC_TurnAngControlpoint2_kph
  Constant7 : Constant  Value=KDSC_TurnAngControlpoint1_deg
  Constant8 : Constant  Value=KDSC_TurnAngControlpoint2_deg
  Constant9 : Constant  Value=KDSC_TurnAngControlpoint2_kph
  Divide1 : Product  Inputs=*/
  Divide8 : Product  Inputs=*/
  Limit : Switch  Criteria=u2 > Threshold  Threshold=KDSC_TurnAngControlpoint1_deg
  Limit1 : Switch  Criteria=u2 > Threshold  Threshold=KDSC_TurnAngControlpoint2_deg
  LowerLimit:10 UpperLimit:Variable : simulink/Discontinuities/Saturation Dynamic  OutMin=[]  OutMax=[]  OutDataTypeStr=Inherit: Same as second input  OutDataType=fixdt(1, 16)  OutScaling=2^-10  DoSatur=off
  Product1 : Product
  Product7 : Product
  VDSC_TurningTargetSpeed : Outport
  wires:
  Divide8/1 -> Product7/2  "Slope"
  [VINP_SASAngle_deg] -> Limit/2
  Add4/1 -> Divide8/2
  Add5/1 -> Divide8/1
  Product7/1 -> Add7/1
  Constant18/1 -> Add5/2
  Constant20/1 -> Add5/1
  Constant12/1 -> Add4/1
  Add6/1 -> Product7/1
  Constant11/1 -> Add4/2
  Constant1/1 -> Add7/2
  Constant4/1 -> Add6/2
  VINP_SASAngle_deg/1 -> [VINP_SASAngle_deg]  "VINP_SASAngle_deg"
  [VINP_SASAngle_deg] -> Add6/1
  VDSC_TurnLimitSpeed_kph/1 -> [VDSC_TurnLimitSpeed_kph]
  [VDSC_TurnLimitSpeed_kph] -> LowerLimit:10 UpperLimit:Variable/1
  Constant2/1 -> LowerLimit:10 UpperLimit:Variable/3
  LowerLimit:10 UpperLimit:Variable/1 -> VDSC_TurningTargetSpeed/1
  Add3/1 -> Product1/1
  Product1/1 -> Add8/1
  [VINP_SASAngle_deg] -> Add3/1
  Constant9/1 -> Limit1/1
  Add1/1 -> Divide1/2
  Constant14/1 -> Add3/2
  Divide1/1 -> Product1/2  "Slope"
  [VINP_SASAngle_deg] -> Limit1/2
  Add2/1 -> Divide1/1
  Constant5/1 -> Add8/2
  Constant7/1 -> Add1/2
  Constant10/1 -> Add2/2
  Constant8/1 -> Add1/1
  Constant6/1 -> Add2/1
  Limit1/1 -> LowerLimit:10 UpperLimit:Variable/2
  Add7/1 -> Limit/3
  Add8/1 -> Limit/1
  Limit/1 -> Limit1/3

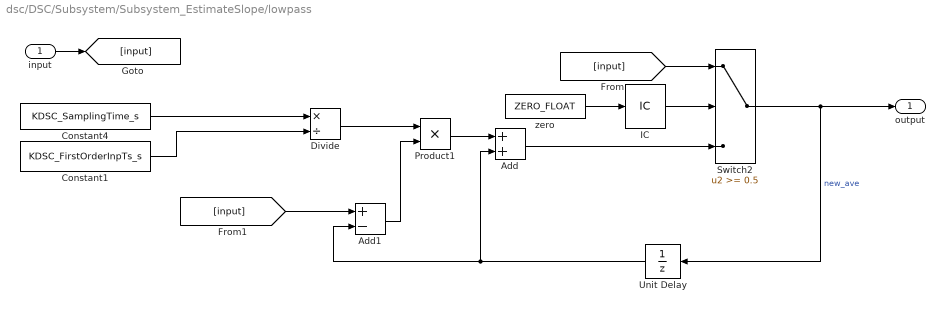
== system dsc/DSC/Subsystem/Subsystem_EstimateSlope/lowpass ==
  input : Inport
  Add : Sum
  Add1 : Sum  Inputs=+-
  Constant1 : Constant  Value=KDSC_FirstOrderInpTs_s  OutDataTypeStr=single
  Constant4 : Constant  Value=KDSC_SamplingTime_s  OutDataTypeStr=single
  Divide : Product  Inputs=*/
  IC : InitialCondition
  Product1 : Product  RndMeth=Zero
  Switch2 : Switch  Tag=struct('comment',struct('text','','placement',1),'logdata',struct('maxnumvals',inf,'plotchannels',[],'stepsize',0,'downsampling',1,'loggingmode',3,'channels',1),'output',struct('width',1,'name','$S_$B','unit','','type','Int32Bin15','offset',0,'max',65535,'min',-65536,'freeze',1,'lsb',2^-15,'arb',0,'class','default','address','','description','','autoscalingmode',1,'lowerheadroom',1,'upperheadroom',1,'headroomunit','bit','checkmin',0,'checkmax',0,'show',0),'threshold',struct('width',1,'name','$S_$B_threshold','unit','','type','Int16','offset',0,'max',NaN,'min',NaN,'freeze',1,'lsb',1,'arb',0,'class','default','address','','description','','value','1','scalar',0),'date',731455.58657044)  Threshold=0.5  InputSameDT=on
  Unit Delay : UnitDelay  SampleTime=-1  HasFrameUpgradeWarning=on
  zero : Constant  Tag=struct('comment',struct('text','','placement',1),'output',struct('width',1,'name','$S_$B','unit','','type','Int16','offset',0,'max',NaN,'min',NaN,'freeze',1,'lsb',1,'arb',0,'class','default','address','','description','','value','0','tolerance',1,'show',0),'date',731455.58675544)  Value=ZERO_FLOAT  OutDataTypeStr=Inherit: Inherit via back propagation
  output : Outport
  wires:
  Add1/1 -> Product1/2
  Product1/1 -> Add/1
  Unit Delay/1 -> Add1/2, Add/2
  Constant4/1 -> Divide/1
  Add/1 -> Switch2/3
  Divide/1 -> Product1/1
  Constant1/1 -> Divide/2
  zero/1 -> IC/1
  IC/1 -> Switch2/2
  Switch2/1 -> output/1, Unit Delay/1  "new_ave"
  input/1 -> [input]
  [input] -> Switch2/1
  [input] -> Add1/1

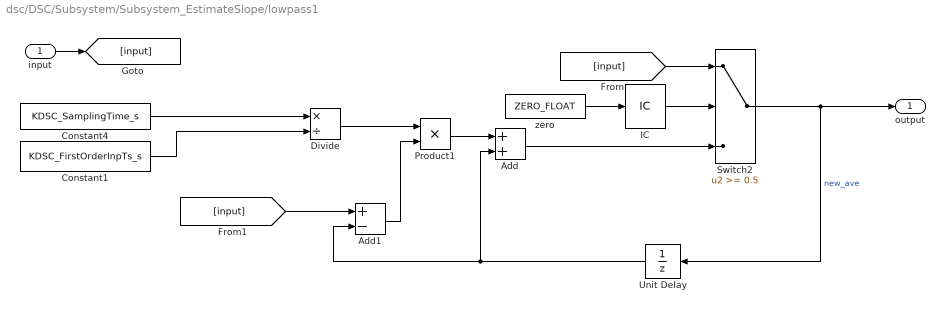
== system dsc/DSC/Subsystem/Subsystem_EstimateSlope/lowpass1 ==
  input : Inport
  Add : Sum
  Add1 : Sum  Inputs=+-
  Constant1 : Constant  Value=KDSC_FirstOrderInpTs_s  OutDataTypeStr=single
  Constant4 : Constant  Value=KDSC_SamplingTime_s  OutDataTypeStr=single
  Divide : Product  Inputs=*/
  IC : InitialCondition
  Product1 : Product  RndMeth=Zero
  Switch2 : Switch  Tag=struct('comment',struct('text','','placement',1),'logdata',struct('maxnumvals',inf,'plotchannels',[],'stepsize',0,'downsampling',1,'loggingmode',3,'channels',1),'output',struct('width',1,'name','$S_$B','unit','','type','Int32Bin15','offset',0,'max',65535,'min',-65536,'freeze',1,'lsb',2^-15,'arb',0,'class','default','address','','description','','autoscalingmode',1,'lowerheadroom',1,'upperheadroom',1,'headroomunit','bit','checkmin',0,'checkmax',0,'show',0),'threshold',struct('width',1,'name','$S_$B_threshold','unit','','type','Int16','offset',0,'max',NaN,'min',NaN,'freeze',1,'lsb',1,'arb',0,'class','default','address','','description','','value','1','scalar',0),'date',731455.58657044)  Threshold=0.5  InputSameDT=on
  Unit Delay : UnitDelay  SampleTime=-1  HasFrameUpgradeWarning=on
  zero : Constant  Tag=struct('comment',struct('text','','placement',1),'output',struct('width',1,'name','$S_$B','unit','','type','Int16','offset',0,'max',NaN,'min',NaN,'freeze',1,'lsb',1,'arb',0,'class','default','address','','description','','value','0','tolerance',1,'show',0),'date',731455.58675544)  Value=ZERO_FLOAT  OutDataTypeStr=Inherit: Inherit via back propagation
  output : Outport
  wires:
  Add1/1 -> Product1/2
  Product1/1 -> Add/1
  Unit Delay/1 -> Add1/2, Add/2
  Constant4/1 -> Divide/1
  Add/1 -> Switch2/3
  Divide/1 -> Product1/1
  Constant1/1 -> Divide/2
  zero/1 -> IC/1
  IC/1 -> Switch2/2
  Switch2/1 -> output/1, Unit Delay/1  "new_ave"
  input/1 -> [input]
  [input] -> Switch2/1
  [input] -> Add1/1

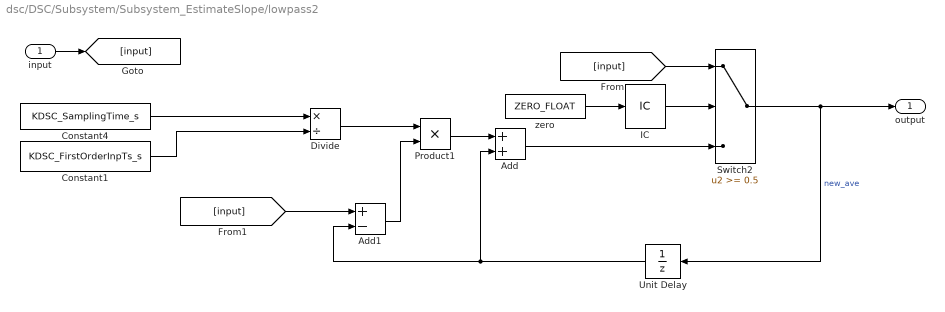
== system dsc/DSC/Subsystem/Subsystem_EstimateSlope/lowpass2 ==
  input : Inport
  Add : Sum
  Add1 : Sum  Inputs=+-
  Constant1 : Constant  Value=KDSC_FirstOrderInpTs_s  OutDataTypeStr=single
  Constant4 : Constant  Value=KDSC_SamplingTime_s  OutDataTypeStr=single
  Divide : Product  Inputs=*/
  IC : InitialCondition
  Product1 : Product  RndMeth=Zero
  Switch2 : Switch  Tag=struct('comment',struct('text','','placement',1),'logdata',struct('maxnumvals',inf,'plotchannels',[],'stepsize',0,'downsampling',1,'loggingmode',3,'channels',1),'output',struct('width',1,'name','$S_$B','unit','','type','Int32Bin15','offset',0,'max',65535,'min',-65536,'freeze',1,'lsb',2^-15,'arb',0,'class','default','address','','description','','autoscalingmode',1,'lowerheadroom',1,'upperheadroom',1,'headroomunit','bit','checkmin',0,'checkmax',0,'show',0),'threshold',struct('width',1,'name','$S_$B_threshold','unit','','type','Int16','offset',0,'max',NaN,'min',NaN,'freeze',1,'lsb',1,'arb',0,'class','default','address','','description','','value','1','scalar',0),'date',731455.58657044)  Threshold=0.5  InputSameDT=on
  Unit Delay : UnitDelay  SampleTime=-1  HasFrameUpgradeWarning=on
  zero : Constant  Tag=struct('comment',struct('text','','placement',1),'output',struct('width',1,'name','$S_$B','unit','','type','Int16','offset',0,'max',NaN,'min',NaN,'freeze',1,'lsb',1,'arb',0,'class','default','address','','description','','value','0','tolerance',1,'show',0),'date',731455.58675544)  Value=ZERO_FLOAT  OutDataTypeStr=Inherit: Inherit via back propagation
  output : Outport
  wires:
  Add1/1 -> Product1/2
  Product1/1 -> Add/1
  Unit Delay/1 -> Add1/2, Add/2
  Constant4/1 -> Divide/1
  Add/1 -> Switch2/3
  Divide/1 -> Product1/1
  Constant1/1 -> Divide/2
  zero/1 -> IC/1
  IC/1 -> Switch2/2
  Switch2/1 -> output/1, Unit Delay/1  "new_ave"
  input/1 -> [input]
  [input] -> Switch2/1
  [input] -> Add1/1

== stateflow chart dsc/DSC/Subsystem/Subsystem_StateSwitch/Chart1 ==
  state DISC_Decide
    state DISC_DISABLED
      VDSC_DISCSta_enum = ENUM_DISCSTA_Disabled;
    state DISC_ENABLED
      state DISC_ON
        state DISC_STANDBY
          VDSC_DISCSta_enum = ENUM_DISCSTA_STANDBY;
        state DISC_ACTIVE
          en:
          VDSC_DISCSta_enum = ENUM_DISCSTA_ACTIVE;
          VDSC_DISCActing_flg= TRUE;
          VDSC_DISCLow_flg =TRUE;
          ex:
          VDSC_DISCActing_flg = FALSE;
          VDSC_DISCLow_flg = FALSE;
          state NoTurnSpdMODE
            VDSC_DISCTurn_flg = FALSE;
          state TurnSpdMODE
            VDSC_DISCTurn_flg=TRUE;
          (default) -> NoTurnSpdMODE
          TurnSpdMODE -> NoTurnSpdMODE : [VDSC_DISCNotTurnReq_flg]
          NoTurnSpdMODE -> TurnSpdMODE : [VDSC_DISCTurnReq_flg]
        (default) -> DISC_STANDBY
        DISC_STANDBY -> DISC_ACTIVE : [VDSC_DISCActiveReq_flg]
        DISC_ACTIVE -> DISC_STANDBY : [!VDSC_DISCActiveReq_flg]
      state DISC_AUTOMODE
        VDSC_DISCSta_enum = ENUM_DISCSTA_OFF;
      (default) -> DISC_AUTOMODE
      DISC_AUTOMODE -> DISC_ON : [VDSC_DISCButtSta_flg]
      DISC_ON -> DISC_AUTOMODE : [!VDSC_DISCButtSta_flg]
    (default) -> DISC_ENABLED
    DISC_DISABLED -> DISC_ENABLED : [VDSC_DISCEnableReq_flg]
    DISC_ENABLED -> DISC_DISABLED : [!VDSC_DISCEnableReq_flg]
  (default) -> DISC_Decide
  data: VDSC_DISCEnableReq_flg input; VDSC_DISCSta_enum output uint8; TRUE parameter; FALSE parameter; VDSC_DISCActiveReq_flg input; VDSC_DISCTurnReq_flg input; VDSC_DISCNotTurnReq_flg input; VDSC_DISCButtSta_flg input; VDSC_DISCTurn_flg output boolean; VDSC_DISCLow_flg output boolean; VDSC_DISCActing_flg output boolean; ENUM_DISCSTA_Disabled parameter; ENUM_DISCSTA_ACTIVE parameter; ENUM_DISCSTA_OFF parameter; ENUM_DISCSTA_STANDBY parameter

== stateflow chart dsc/DSC/Subsystem/Subsystem_ComtrolSpd/Chart ==
  state inactive
    VDSC_ModeSwitch_flg=FALSE
  state avtive
    VDSC_ModeSwitch_flg=TRUE;
  (default) -> inactive
  inactive -> avtive : [VDISC_DISCTurn_flg == 1]
  avtive -> inactive : [VVMC_MeterIndSpeedForCalcu_kph > VDSC_TurnLimitSpeed_kph && VDISC_DISCTurn_flg  ~= 1]
  data: VVMC_MeterIndSpeedForCalcu_kph input; VDSC_ModeSwitch_flg output boolean; VDSC_TurnLimitSpeed_kph input; VDISC_DISCTurn_flg input; TRUE parameter; FALSE parameter

== stateflow chart dsc/DSC/Subsystem/Subsystem_AutoMode/Mode ==
  state DISCSta_OFF
    VDSC_DISCButtSta_flg = 0;
  state DISCSta_ON
    VDSC_DISCButtSta_flg = 1;
  (default) -> DISCSta_OFF
  DISCSta_OFF -> DISCSta_ON : [VDSC_DISCButtReq_flg ==1]
  DISCSta_ON -> DISCSta_OFF : [VDSC_DISCButtReq_flg ==1]
  data: VDSC_DISCButtReq_flg input; VDSC_DISCButtSta_flg output double

== stateflow chart dsc/DSC/Subsystem/Subsystem_TempWarning/Chart1 ==
  state DISC_NoWarning
    VDSC_TempWarning_flg = FALSE;
  state DISC_Warning
    VDSC_TempWarning_flg = TRUE;
  (default) -> DISC_NoWarning
  DISC_NoWarning -> DISC_Warning : [VINP_BrkDiscTempSta_enum == 1 ]
  DISC_Warning -> DISC_NoWarning : [VINP_BrkDiscTempSta_enum  == 0  ]
  data: VINP_BrkDiscTempSta_enum input; FALSE parameter; TRUE parameter; VDSC_TempWarning_flg output boolean
